simulink model "gm_resource_sharing_multi_module_phase_shift_generator_base"  (R2025b)
settings: Solver=FixedStepDiscrete  StartTime=0.0  StopTime=10e3  RelTol=1e-3
libraries: simulink x2, simulink_need_slupdate x1, hdlsllib x1
settings Model: Creator=KoayXianCong  LastModifiedBy=KoayXianCong
settings OptimizationCC: BlockReduction=off  ConditionallyExecuteInputs=off  DefaultParameterBehavior=Inlined  InheritOutputTypeSmallerThanSingle=on
settings DebuggingCC: SignalRangeChecking=warning  ArtificialAlgebraicLoopMsg=error  InheritedTsInSrcMsg=none  SingleTaskRateTransMsg=error
settings HardwareCC: ProdBitPerPointer=32.0  ProdBitPerSizeT=32.0  ProdBitPerPtrDiffT=32.0  ProdLargestAtomicFloat=None  ProdIntDivRoundTo=Undefined  ProdEndianess=Unspecified  ProdWordSize=32.0  ProdHWDeviceType=ASIC/FPGA->ASIC/FPGA  TargetBitPerPointer=64.0  TargetBitPerSizeT=64.0  TargetBitPerPtrDiffT=64.0  TargetLongLongMode=on  TargetIntDivRoundTo=Zero  TargetEndianess=LittleEndian  TargetWordSize=64.0  TargetHWDeviceType=Custom Processor->MATLAB Host Computer  ProdEqTarget=off

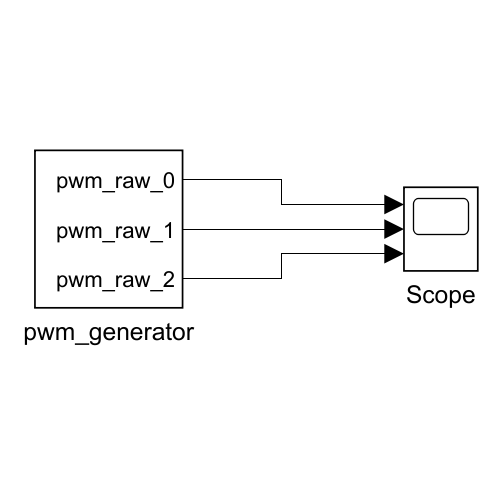
[thumbnail: Simulink's stored preview of the top-level diagram]
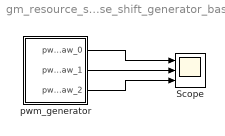
== system gm_resource_sharing_multi_module_phase_shift_generator_base ==
  Scope : Scope  NumInputPorts=3
      settings: ActiveDisplayYMinimum=-0.12499999999999997  ActiveDisplayYMaximum=1.125
  pwm_generator : Subsystem
  wires:
  pwm_generator/3(pwm_raw_2) -> Scope/3
  pwm_generator/2(pwm_raw_1) -> Scope/2
  pwm_generator/1(pwm_raw_0) -> Scope/1

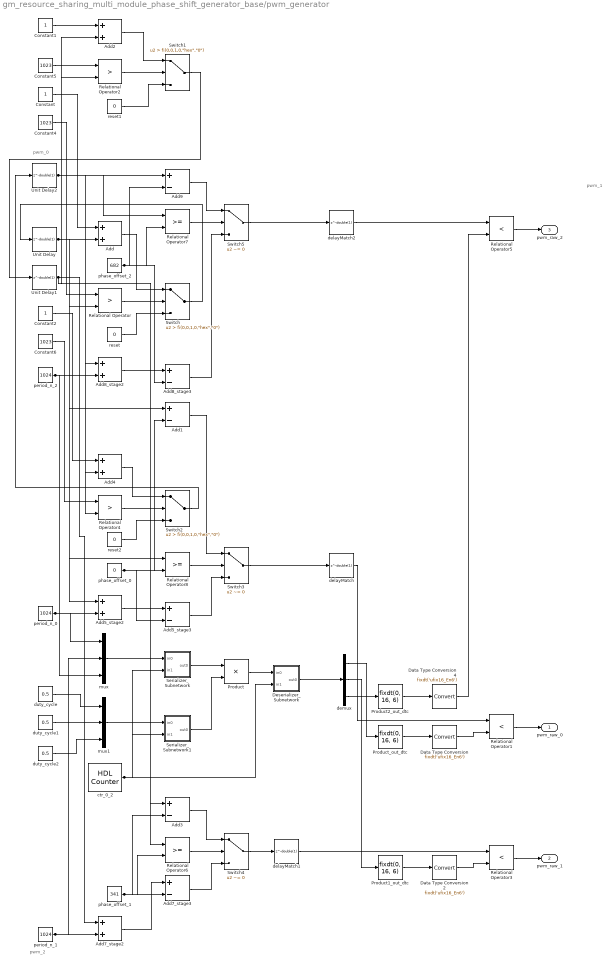
== system gm_resource_sharing_multi_module_phase_shift_generator_base/pwm_generator ==
  note: pwm_0
  note: pwm_1
  note: pwm_2
  Add : Sum  OutDataTypeStr=fixdt(0, 16, 5)  AccumDataTypeStr=fixdt(0, 27, 15)  SampleTime=1
  Add1 : Sum  Inputs=+-  OutDataTypeStr=fixdt(1, 18, 5)  AccumDataTypeStr=fixdt(1, 18, 5)  SampleTime=1
  Add2 : Sum  OutDataTypeStr=fixdt(0, 16, 5)  AccumDataTypeStr=fixdt(0, 27, 15)  SampleTime=1
  Add3 : Sum  Inputs=+-  OutDataTypeStr=fixdt(1, 19, 7)  AccumDataTypeStr=fixdt(1, 19, 7)  SampleTime=1
  Add4 : Sum  OutDataTypeStr=fixdt(0, 16, 5)  AccumDataTypeStr=fixdt(0, 27, 15)  SampleTime=1
  Add5_stage2 : Sum  OutDataTypeStr=fixdt(0, 22, 5)  AccumDataTypeStr=fixdt(1, 23, 5)  SampleTime=1
  Add5_stage3 : Sum  Inputs=+-  OutDataTypeStr=fixdt(1, 23, 5)  AccumDataTypeStr=fixdt(1, 23, 5)  SampleTime=1
  Add7_stage2 : Sum  OutDataTypeStr=fixdt(0, 22, 5)  AccumDataTypeStr=fixdt(1, 25, 7)  SampleTime=1
  Add7_stage3 : Sum  Inputs=+-  OutDataTypeStr=fixdt(1, 25, 7)  AccumDataTypeStr=fixdt(1, 25, 7)  SampleTime=1
  Add8_stage2 : Sum  OutDataTypeStr=fixdt(0, 22, 5)  AccumDataTypeStr=fixdt(1, 24, 6)  SampleTime=1
  Add8_stage3 : Sum  Inputs=+-  OutDataTypeStr=fixdt(1, 24, 6)  AccumDataTypeStr=fixdt(1, 24, 6)  SampleTime=1
  Add9 : Sum  Inputs=+-  OutDataTypeStr=fixdt(1, 18, 6)  AccumDataTypeStr=fixdt(1, 18, 6)  SampleTime=1
  Constant : Constant  OutDataTypeStr=fixdt(0, 16, 15)  SampleTime=1
  Constant1 : Constant  OutDataTypeStr=fixdt(0, 16, 15)  SampleTime=1
  Constant2 : Constant  OutDataTypeStr=fixdt(0, 16, 15)  SampleTime=1
  Constant4 : Constant  Value=1023  OutDataTypeStr=uint16  SampleTime=1
  Constant5 : Constant  Value=1023  OutDataTypeStr=uint16  SampleTime=1
  Constant6 : Constant  Value=1023  OutDataTypeStr=uint16  SampleTime=1
  Data Type Conversion : DataTypeConversion  OutDataTypeStr=fixdt('ufix16_En6')
  Data Type Conversion2 : DataTypeConversion  OutDataTypeStr=fixdt('ufix16_En6')
  Data Type Conversion4 : DataTypeConversion  OutDataTypeStr=fixdt('ufix16_En6')
  Deserializer_Subnetwork : Subsystem
  Product : Product  Inputs=**  OutDataTypeStr=fixdt(0, 32, 16)  SampleTime=0.333333333333333
  Product1_out_dtc : DataTypeConversion  OutDataTypeStr=fixdt(0, 16, 6)  SampleTime=1  SaturateOnIntegerOverflow=off  RndMeth=Floor
  Product2_out_dtc : DataTypeConversion  OutDataTypeStr=fixdt(0, 16, 6)  SampleTime=1  SaturateOnIntegerOverflow=off  RndMeth=Floor
  Product_out_dtc : DataTypeConversion  OutDataTypeStr=fixdt(0, 16, 6)  SampleTime=1  SaturateOnIntegerOverflow=off  RndMeth=Floor
  Relational Operator : RelationalOperator  Operator=>  OutDataTypeStr=boolean  SampleTime=1  InputSameDT=off
  Relational Operator1 : RelationalOperator  Operator=<  OutDataTypeStr=boolean  SampleTime=1  InputSameDT=off
  Relational Operator2 : RelationalOperator  Operator=>  OutDataTypeStr=boolean  SampleTime=1  InputSameDT=off
  Relational Operator3 : RelationalOperator  Operator=<  OutDataTypeStr=boolean  SampleTime=1  InputSameDT=off
  Relational Operator4 : RelationalOperator  Operator=>  OutDataTypeStr=boolean  SampleTime=1  InputSameDT=off
  Relational Operator5 : RelationalOperator  Operator=<  OutDataTypeStr=boolean  SampleTime=1  InputSameDT=off
  Relational Operator6 : RelationalOperator  OutDataTypeStr=boolean  SampleTime=1  InputSameDT=off
  Relational Operator7 : RelationalOperator  OutDataTypeStr=boolean  SampleTime=1  InputSameDT=off
  Relational Operator8 : RelationalOperator  OutDataTypeStr=boolean  SampleTime=1  InputSameDT=off
  Serializer_Subnetwork : Subsystem
  Serializer_Subnetwork1 : Subsystem
  Switch : Switch  Criteria=u2 > Threshold  Threshold="fi(0,0,1,0,\"hex\",\"0\")"  OutDataTypeStr=fixdt(0, 16, 5)  SampleTime=1  SaturateOnIntegerOverflow=off  InputSameDT=off
  Switch1 : Switch  Criteria=u2 > Threshold  Threshold="fi(0,0,1,0,\"hex\",\"0\")"  OutDataTypeStr=fixdt(0, 16, 5)  SampleTime=1  SaturateOnIntegerOverflow=off  InputSameDT=off
  Switch2 : Switch  Criteria=u2 > Threshold  Threshold="fi(0,0,1,0,\"hex\",\"0\")"  OutDataTypeStr=fixdt(0, 16, 5)  SampleTime=1  SaturateOnIntegerOverflow=off  InputSameDT=off
  Switch3 : Switch  Criteria=u2 ~= 0  Threshold="fi(0,0,1,0,\"hex\",\"0\")"  OutDataTypeStr=fixdt(1, 23, 5)  SampleTime=1  SaturateOnIntegerOverflow=off  InputSameDT=off
  Switch4 : Switch  Criteria=u2 ~= 0  Threshold="fi(0,0,1,0,\"hex\",\"0\")"  OutDataTypeStr=fixdt(1, 25, 7)  SampleTime=1  SaturateOnIntegerOverflow=off  InputSameDT=off
  Switch5 : Switch  Criteria=u2 ~= 0  Threshold="fi(0,0,1,0,\"hex\",\"0\")"  OutDataTypeStr=fixdt(1, 24, 6)  SampleTime=1  SaturateOnIntegerOverflow=off  InputSameDT=off
  Unit Delay : Delay  DelayLength=double(1)  InitialCondition=0  SampleTime=1
  Unit Delay1 : Delay  DelayLength=double(1)  InitialCondition=0  SampleTime=1
  Unit Delay2 : Delay  DelayLength=double(1)  InitialCondition=0  SampleTime=1
  ctr_0_2 : hdlsllib/Sources/HDL Counter  CountType=Count limited  CountInit=double(0)  CountStep=double(1)  CountMax=double(2)  CountFromType=Initial value  CountFrom=double(0)  CountResetPort=off  CountLoadPort=off  CountEnbPort=off  CountDirPort=off  CountHitOutputPort=off  CountDataType=Unsigned  CountWordLen=2  CountFracLen=0  CountSampTime=0.333333333333333
  delayMatch : Delay  DelayLength=double(1)  InitialCondition=0  SampleTime=1
  delayMatch1 : Delay  DelayLength=double(1)  InitialCondition=0  SampleTime=1
  delayMatch2 : Delay  DelayLength=double(1)  InitialCondition=0  SampleTime=1
  demux : Demux  Outputs=3
  duty_cycle : Constant  Value=0.5  OutDataTypeStr=fixdt(0, 16, 16)  SampleTime=1
  duty_cycle1 : Constant  Value=0.5  OutDataTypeStr=fixdt(0, 16, 16)  SampleTime=1
  duty_cycle2 : Constant  Value=0.5  OutDataTypeStr=fixdt(0, 16, 16)  SampleTime=1
  mux : Mux  Inputs=3
  mux1 : Mux  Inputs=3
  period_n_0 : Constant  Value=1024  OutDataTypeStr=uint16  SampleTime=1
  period_n_1 : Constant  Value=1024  OutDataTypeStr=uint16  SampleTime=1
  period_n_2 : Constant  Value=1024  OutDataTypeStr=uint16  SampleTime=1
  phase_offset_0 : Constant  Value=0  OutDataTypeStr=fixdt(1, 16, 4)  SampleTime=1
  phase_offset_1 : Constant  Value=341  OutDataTypeStr=fixdt(0, 16, 7)  SampleTime=1
  phase_offset_2 : Constant  Value=682  OutDataTypeStr=fixdt(0, 16, 6)  SampleTime=1
  reset : Constant  Value=0  OutDataTypeStr=fixdt(1, 16, 4)  SampleTime=1
  reset1 : Constant  Value=0  OutDataTypeStr=fixdt(1, 16, 4)  SampleTime=1
  reset2 : Constant  Value=0  OutDataTypeStr=fixdt(1, 16, 4)  SampleTime=1
  pwm_raw_0 : Outport  SampleTime=1
  pwm_raw_1 : Outport  Port=2  SampleTime=1
  pwm_raw_2 : Outport  Port=3  SampleTime=1
  wires:
  Unit Delay1/1 -> Relational Operator6/1, Add3/1, Add7_stage2/1, Add2/2, Relational Operator2/2
  Unit Delay/1 -> Relational Operator8/1, Add1/1, Add5_stage2/1, Add/2, Relational Operator/2
  Constant6/1 -> Relational Operator4/1
  Unit Delay2/1 -> Relational Operator7/1, Add8_stage2/1, Add9/1, Relational Operator4/2, Add4/2
  Constant1/1 -> Add2/1
  demux/2 -> Product1_out_dtc/1
  duty_cycle2/1 -> mux1/3
  demux/1 -> Product_out_dtc/1
  Constant5/1 -> Relational Operator2/1
  Constant/1 -> Add/1
  mux/1 -> Serializer_Subnetwork/1(in0)
  mux1/1 -> Serializer_Subnetwork1/1(in0)
  Constant4/1 -> Relational Operator/1
  Constant2/1 -> Add4/1
  period_n_2/1 -> Add8_stage2/2, mux/3
  period_n_0/1 -> mux/1, Add5_stage2/2
  demux/3 -> Product2_out_dtc/1
  Add8_stage3/1 -> Switch5/3
  Data Type Conversion2/1 -> Relational Operator3/2
  duty_cycle/1 -> mux1/1
  duty_cycle1/1 -> mux1/2
  Relational Operator6/1 -> Switch4/2
  delayMatch/1 -> Relational Operator1/1
  period_n_1/1 -> Add7_stage2/2, mux/2
  Add5_stage2/1 -> Add5_stage3/1
  Add2/1 -> Switch1/1
  Relational Operator2/1 -> Switch1/2
  reset1/1 -> Switch1/3
  Add/1 -> Switch/1
  phase_offset_2/1 -> Relational Operator7/2, Add8_stage3/2, Add9/2
  Relational Operator/1 -> Switch/2
  Relational Operator3/1 -> pwm_raw_1/1
  reset/1 -> Switch/3
  Add8_stage2/1 -> Add8_stage3/1
  Data Type Conversion/1 -> Relational Operator1/2
  Add4/1 -> Switch2/1
  Relational Operator4/1 -> Switch2/2
  reset2/1 -> Switch2/3
  phase_offset_0/1 -> Relational Operator8/2, Add5_stage3/2, Add1/2
  delayMatch1/1 -> Relational Operator3/1
  Switch4/1 -> delayMatch1/1
  ctr_0_2/1 -> Deserializer_Subnetwork/2(in1), Serializer_Subnetwork/2(in1), Serializer_Subnetwork1/2(in1)
  delayMatch2/1 -> Relational Operator5/1
  phase_offset_1/1 -> Add7_stage3/2, Add3/2, Relational Operator6/2
  Add7_stage2/1 -> Add7_stage3/1
  Switch1/1 -> Unit Delay1/1
  Switch5/1 -> delayMatch2/1
  Add9/1 -> Switch5/1
  Relational Operator7/1 -> Switch5/2
  Switch/1 -> Unit Delay/1
  Add1/1 -> Switch3/1
  Switch2/1 -> Unit Delay2/1
  Relational Operator8/1 -> Switch3/2
  Add5_stage3/1 -> Switch3/3
  Product1_out_dtc/1 -> Data Type Conversion2/1
  Add7_stage3/1 -> Switch4/3
  Serializer_Subnetwork/1(out0) -> Product/1
  Serializer_Subnetwork1/1(out0) -> Product/2
  Add3/1 -> Switch4/1
  Switch3/1 -> delayMatch/1
  Product/1 -> Deserializer_Subnetwork/1(in0)
  Deserializer_Subnetwork/1(out0) -> demux/1
  Product2_out_dtc/1 -> Data Type Conversion4/1
  Product_out_dtc/1 -> Data Type Conversion/1
  Data Type Conversion4/1 -> Relational Operator5/2
  Relational Operator5/1 -> pwm_raw_2/1
  Relational Operator1/1 -> pwm_raw_0/1

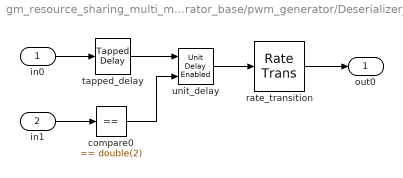
== system gm_resource_sharing_multi_module_phase_shift_generator_base/pwm_generator/Deserializer_Subnetwork ==
  in0 : Inport  OutDataTypeStr=fixdt(0, 32, 16)  SampleTime=0.333333333333333
  in1 : Inport  Port=2  OutDataTypeStr=fixdt(0, 2, 0)  SampleTime=0.333333333333333
  compare0 : simulink/Logic and Bit Operations/Compare To Constant  relop===  const=double(2)  OutDataTypeStr=boolean
  rate_transition : RateTransition  Integrity=off  Deterministic=off  OutPortSampleTimeOpt=Multiple of input port sample time  OutPortSampleTimeMultiple=3
  tapped_delay : simulink/Discrete/Tapped Delay  vinit=0  samptime=-1  NumDelays=double(2)  DelayOrder=Oldest  includeCurrent=on
  unit_delay : simulink_need_slupdate/Unit Delay Enabled  vinit=0.0  tsamp=-1
  out0 : Outport  OutDataTypeStr=fixdt(0, 32, 16)  PortDimensions=[3]  SampleTime=1
  wires:
  unit_delay/1 -> rate_transition/1
  in0/1 -> tapped_delay/1
  in1/1 -> compare0/1
  tapped_delay/1 -> unit_delay/1
  compare0/1 -> unit_delay/2
  rate_transition/1 -> out0/1

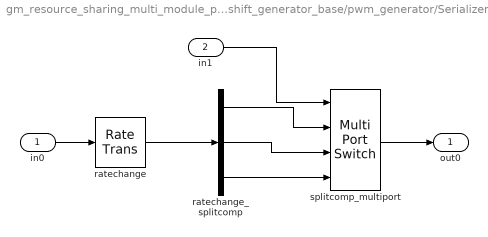
== system gm_resource_sharing_multi_module_phase_shift_generator_base/pwm_generator/Serializer_Subnetwork ==
  in0 : Inport  OutDataTypeStr=uint16  PortDimensions=[3]  SampleTime=1
  in1 : Inport  Port=2  OutDataTypeStr=fixdt(0, 2, 0)  SampleTime=0.333333333333333
  ratechange : RateTransition  Integrity=off  Deterministic=off  OutPortSampleTimeOpt=Multiple of input port sample time  OutPortSampleTimeMultiple=1/3
  ratechange_splitcomp : Demux  Outputs=3
  splitcomp_multiport : MultiPortSwitch  DataPortOrder=Zero-based contiguous  DiagnosticForDefault=None  zeroidx=on  OutDataTypeStr=uint16  SampleTime=0.333333333333333  SaturateOnIntegerOverflow=off  InputSameDT=off
  out0 : Outport  OutDataTypeStr=uint16  SampleTime=0.333333333333333
  wires:
  splitcomp_multiport/1 -> out0/1
  in0/1 -> ratechange/1
  ratechange/1 -> ratechange_splitcomp/1
  in1/1 -> splitcomp_multiport/1
  ratechange_splitcomp/1 -> splitcomp_multiport/2
  ratechange_splitcomp/3 -> splitcomp_multiport/4
  ratechange_splitcomp/2 -> splitcomp_multiport/3

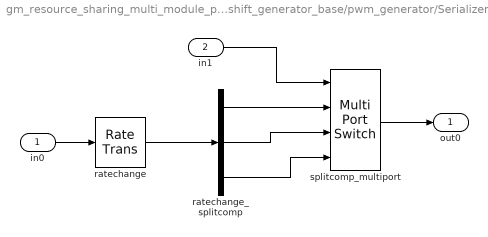
== system gm_resource_sharing_multi_module_phase_shift_generator_base/pwm_generator/Serializer_Subnetwork1 ==
  in0 : Inport  OutDataTypeStr=fixdt(0, 16, 16)  PortDimensions=[3]  SampleTime=1
  in1 : Inport  Port=2  OutDataTypeStr=fixdt(0, 2, 0)  SampleTime=0.333333333333333
  ratechange : RateTransition  Integrity=off  Deterministic=off  OutPortSampleTimeOpt=Multiple of input port sample time  OutPortSampleTimeMultiple=1/3
  ratechange_splitcomp : Demux  Outputs=3
  splitcomp_multiport : MultiPortSwitch  DataPortOrder=Zero-based contiguous  DiagnosticForDefault=None  zeroidx=on  OutDataTypeStr=fixdt(0, 16, 16)  SampleTime=0.333333333333333  SaturateOnIntegerOverflow=off  InputSameDT=off
  out0 : Outport  OutDataTypeStr=fixdt(0, 16, 16)  SampleTime=0.333333333333333
  wires:
  in0/1 -> ratechange/1
  ratechange/1 -> ratechange_splitcomp/1
  in1/1 -> splitcomp_multiport/1
  ratechange_splitcomp/2 -> splitcomp_multiport/3
  ratechange_splitcomp/1 -> splitcomp_multiport/2
  ratechange_splitcomp/3 -> splitcomp_multiport/4
  splitcomp_multiport/1 -> out0/1
